simulink library "sunsensor2body_lib1"  (R2018b)
settings: Solver=VariableStepAuto  StartTime=0.0  StopTime=10.0  RelTol=1e-3
undefined symbols (not defined in the file or in its folder): simParams
libraries: aerolibutil x1
settings Model: Creator=kylle  LastModifiedBy=kylle

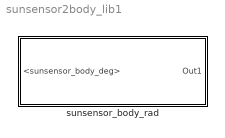
== system sunsensor2body_lib1 ==
  sunsensor_body_rad : Subsystem

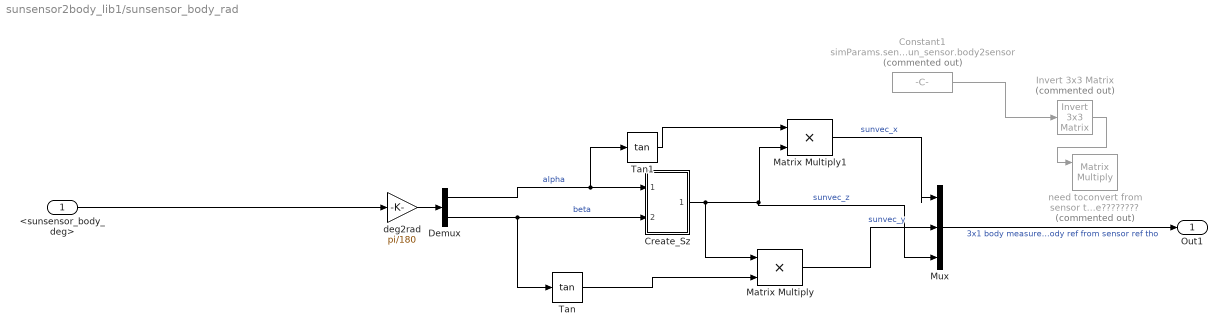
== system sunsensor2body_lib1/sunsensor_body_rad ==
  <sunsensor_body_deg> : Inport
  Constant1 : Constant  Commented=on  Value=simParams.sensors.sun_sensor.body2sensor
  Create_Sz : Subsystem
  Demux : Demux  Outputs=2
  Invert 3x3 Matrix : aerolibutil/Invert  3x3 Matrix  Commented=on
  Matrix Multiply : Product
  Matrix Multiply1 : Product
  Mux : Mux  Inputs=3
  Tan : Trigonometry  Operator=tan
  Tan1 : Trigonometry  Operator=tan
  deg2rad : Gain  Gain=pi/180
  need toconvert from sensor to body frame???????? : Product  Commented=on  Multiplication=Matrix(*)
  Out1 : Outport
  wires:
  Tan/1 -> Matrix Multiply/2
  Demux/1 -> Tan1/1, Create_Sz/1(alpha)  "alpha"
  Matrix Multiply/1 -> Mux/2  "sunvec_y"
  Create_Sz/1(Out1) -> Mux/3, Matrix Multiply1/2, Matrix Multiply/1  "sunvec_z"
  Demux/2 -> Tan/1, Create_Sz/2(beta)  "beta"
  Tan1/1 -> Matrix Multiply1/1
  deg2rad/1 -> Demux/1
  Matrix Multiply1/1 -> Mux/1  "sunvec_x"
  <sunsensor_body_deg>/1 -> deg2rad/1
  Constant1/1 -> Invert 3x3 Matrix/1
  Invert 3x3 Matrix/1 -> need toconvert from sensor to body frame????????/1
  Mux/1 -> Out1/1  "3x1 body measurements from sun sensor (possibly need to change into body ref from sensor ref tho"

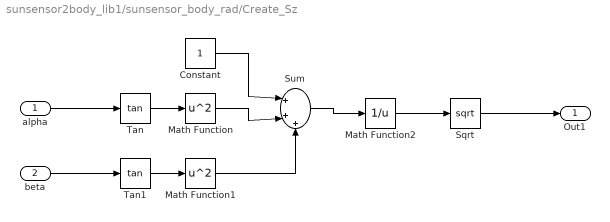
== system sunsensor2body_lib1/sunsensor_body_rad/Create_Sz ==
  alpha : Inport
  beta : Inport  Port=2
  Constant : Constant
  Math Function : Math  Operator=square  SaturateOnIntegerOverflow=on
  Math Function1 : Math  Operator=square  SaturateOnIntegerOverflow=on
  Math Function2 : Math  Operator=reciprocal  SaturateOnIntegerOverflow=on
  Sqrt : Sqrt  SaturateOnIntegerOverflow=on
  Sum : Sum  Inputs=|+++
  Tan : Trigonometry  Operator=tan
  Tan1 : Trigonometry  Operator=tan
  Out1 : Outport
  wires:
  Constant/1 -> Sum/1
  Sum/1 -> Math Function2/1
  Tan/1 -> Math Function/1
  Math Function/1 -> Sum/2
  Math Function2/1 -> Sqrt/1
  Tan1/1 -> Math Function1/1
  alpha/1 -> Tan/1
  beta/1 -> Tan1/1
  Math Function1/1 -> Sum/3
  Sqrt/1 -> Out1/1
